simulink model "Zamora22210432HIPER"  (R2023a)
settings: Solver=ode15s  StartTime=0.0  StopTime=15  RelTol=1e-3
libraries: slpidlib x1
settings Model: Creator=Michelle  LastModifiedBy=Michelle
settings DataIOCC: ReturnWorkspaceOutputs=off  TimeSaveName=t
settings DebuggingCC: AlgebraicLoopMsg=none  ArtificialAlgebraicLoopMsg=none  MaxConsecutiveZCsMsg=none  InheritedTsInSrcMsg=none  MultiTaskCondExecSysMsg=none  MultiTaskRateTransMsg=warning  TasksWithSamePriorityMsg=none  SigSpecEnsureSampleTimeMsg=none  UnknownTsInhSupMsg=none  ModelReferenceExtraNoncontSigs=none  OperatingPointInterfaceChecksumMismatchMsg=none

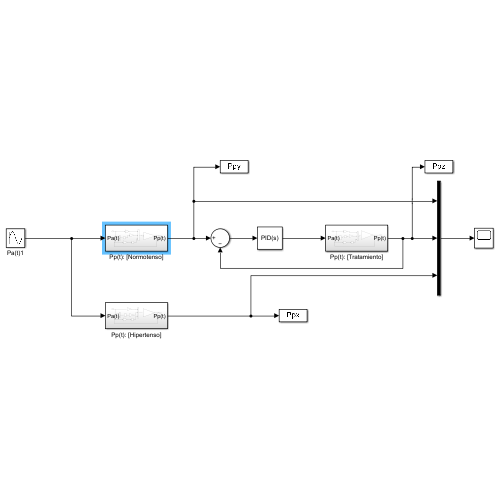
[thumbnail: Simulink's stored preview of the top-level diagram]
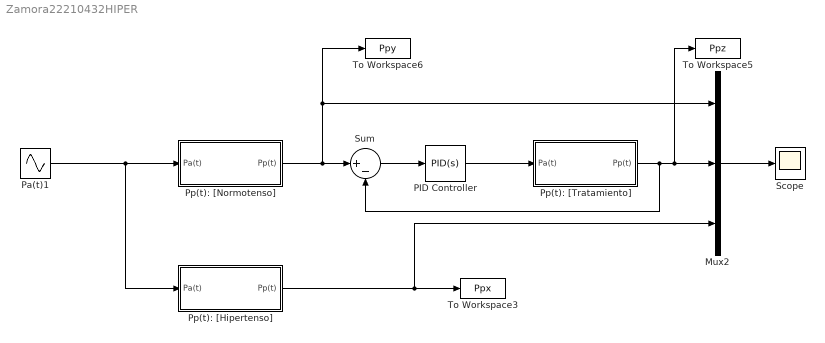
== system Zamora22210432HIPER ==
  Mux2 : Mux  Inputs=3
  PID Controller : slpidlib/PID Controller  Controller=PID  Form=Parallel  TimeDomain=Continuous-time  UseExternalTs=off  SampleTime=-1  IntegratorMethod=Forward Euler  FilterMethod=Forward Euler  ControllerParametersSource=internal  P=8.92851562535347e-05  I=1035.71406250139  UseKiTs=off  D=0  N=100  UseFilter=on  TunerSelectOption=Transfer Function Based (PID Tuner App)  InitialConditionSource=internal  InitialConditionForIntegrator=0  InitialConditionForFilter=0  DifferentiatorICPrevScaledInput=0  ExternalReset=none  TrackingMode=off  Kt=1  LimitOutput=off  SatLimitsSource=internal  UpperSaturationLimit=inf  LowerSaturationLimit=-inf  LinearizeAsGain=on  AntiWindupMode=none  Kb=1  LimitIntegrator=off  UpperIntegratorSaturationLimit=inf  LowerIntegratorSaturationLimit=-inf  POutMin=[]  POutMax=[]  IOutMin=[]  IOutMax=[]  DOutMin=[]  DOutMax=[]  NOutMin=[]  NOutMax=[]  SumOutMin=[]  SumOutMax=[]  SaturationOutMin=[]  SaturationOutMax=[]  PParamMin=[]  PParamMax=[]  IParamMin=[]  IParamMax=[]  DParamMin=[]  DParamMax=[]  NParamMin=[]  NParamMax=[]  KbParamMin=[]  KbParamMax=[]  KtParamMin=[]  KtParamMax=[]  KbOutMin=[]  KbOutMax=[]  KtOutMin=[]  KtOutMax=[]  IntegratorOutMin=[]  IntegratorOutMax=[]  FilterOutMin=[]  FilterOutMax=[]  SumI1OutMin=[]  SumI1OutMax=[]  SumI2OutMin=[]  SumI2OutMax=[]  SumI3OutMin=[]  SumI3OutMax=[]  SumI4OutMin=[]  SumI4OutMax=[]  SumDOutMin=[]  SumDOutMax=[]  DifferentiatorOutMin=[]  DifferentiatorOutMax=[]  FilterDiffOutCoefMin=[]  FilterDiffOutCoefMax=[]  ReciprocalOutMin=[]  ReciprocalOutMax=[]  SumDenOutMin=[]  SumDenOutMax=[]  SumNumOutMin=[]  SumNumOutMax=[]  DivideOutMin=[]  DivideOutMax=[]  UdiffTsProdOutMin=[]  UdiffTsProdOutMax=[]  NTsProdOutMin=[]  NTsProdOutMax=[]  UintegralTsProdOutMin=[]  UintegralTsProdOutMax=[]  UngainTsProdOutMin=[]  UngainTsProdOutMax=[]  ClampingZeroOutDataTypeStr=Inherit: Inherit via back propagation  ClampingZeroOutMin=[]  ClampingZeroOutMax=[]  FilterDenConstantOutDataTypeStr=Inherit: Inherit via back propagation  FilterDenConstantOutMin=[]  FilterDenConstantOutMax=[]  PCopyOutDataTypeStr=Inherit: Inherit via back propagation  PCopyOutMin=[]  PCopyOutMax=[]  NCopyOutDataTypeStr=Inherit: Inherit via back propagation  NCopyOutMin=[]  NCopyOutMax=[]  IntegratorContinuousStateAttributes=''  IntegratorStateMustResolveToSignalObject=off  IntegratorRTWStateStorageClass=Auto  FilterContinuousStateAttributes=''  FilterStateMustResolveToSignalObject=off  FilterRTWStateStorageClass=Auto  ParallelPVariant=InternalParameters  IdealPVariant=Disabled  IVariant=InternalParameters  DVariant=InternalParameters  IntegratorVariant=Continuous  SatVariant=Disabled  AWVariant=Passthrough  PCopyVariant=Disabled  TRVariant=Disabled  FdbkBlocksVariant=Forward  IdealPFdbkVariant=Disabled  SatFdbkVariant=Disabled  DerivativeFilterVariant=ContFilter  NVariant=InternalParameters  NCopyVariant=Disabled  FilterICVariant=InternalICsFilter  IntegratorICVariant=InternalICs  ExternalResetVariant=Disabled  TRSumVariant=Passthrough  SumFdbkVariant=Disabled  SumVariant=Sum_PID  TsampFilterVariant=InternalTs  TsampNgainVariant=Passthrough  TsampIntegralVariant=Disabled_SignalSpec  ExternalSaturationOutDataTypeStr=Inherit: Same as second input
  Pa(t)1 : Sin  Bias=0.8  Frequency=(2*pi)*(95/60)
  Pp(t): [Hipertenso] : Subsystem
  Pp(t): [Normotenso] : Subsystem
  Pp(t): [Tratamiento] : Subsystem
  Scope : Scope
  Sum : Sum  Inputs=|+-
  To Workspace3 : ToWorkspace  VariableName=Ppx  SampleTime=-1
  To Workspace5 : ToWorkspace  VariableName=Ppz  SampleTime=-1
  To Workspace6 : ToWorkspace  VariableName=Ppy  SampleTime=-1
  wires:
  Pp(t): [Tratamiento]/1(Pp(t)) -> Mux2/2, To Workspace5/1, Sum/2
  Mux2/1 -> Scope/1
  Pp(t): [Normotenso]/1(Pp(t)) -> Mux2/1, To Workspace6/1, Sum/1
  Sum/1 -> PID Controller/1
  Pp(t): [Hipertenso]/1(Pp(t)) -> Mux2/3, To Workspace3/1
  Pa(t)1/1 -> Pp(t): [Hipertenso]/1(Pa(t)), Pp(t): [Normotenso]/1(Pa(t))
  PID Controller/1 -> Pp(t): [Tratamiento]/1(Pa(t))

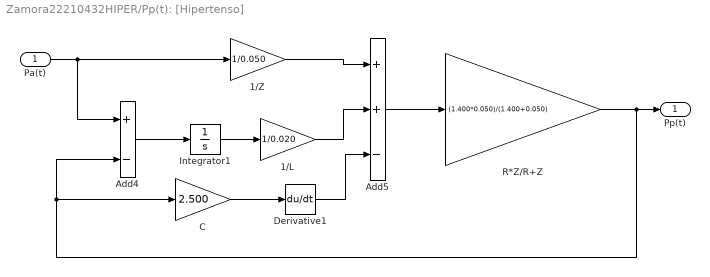
== system Zamora22210432HIPER/Pp(t): [Hipertenso] ==
  Pa(t) : Inport
  1/L : Gain  Gain=1/0.020
  1/Z : Gain  Gain=1/0.050
  Add4 : Sum  Inputs=+-
  Add5 : Sum  Inputs=++-
  C : Gain  Gain=2.500
  Derivative1 : Derivative
  Integrator1 : Integrator
  R*Z/R+Z : Gain  Gain=(1.400*0.050)/(1.400+0.050)
  Pp(t) : Outport  VectorParamsAs1DForOutWhenUnconnected=off
  wires:
  1/Z/1 -> Add5/1
  Derivative1/1 -> Add5/3
  C/1 -> Derivative1/1
  Add5/1 -> R*Z/R+Z/1
  Pa(t)/1 -> Add4/1, 1/Z/1
  R*Z/R+Z/1 -> C/1, Add4/2, Pp(t)/1
  Add4/1 -> Integrator1/1
  Integrator1/1 -> 1/L/1
  1/L/1 -> Add5/2

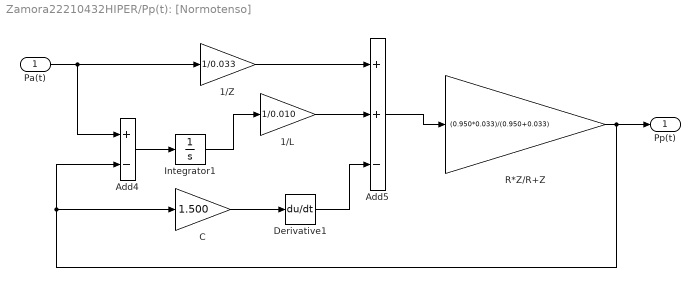
== system Zamora22210432HIPER/Pp(t): [Normotenso] ==
  Pa(t) : Inport
  1/L : Gain  Gain=1/0.010
  1/Z : Gain  Gain=1/0.033
  Add4 : Sum  Inputs=+-
  Add5 : Sum  Inputs=++-
  C : Gain  Gain=1.500
  Derivative1 : Derivative
  Integrator1 : Integrator
  R*Z/R+Z : Gain  Gain=(0.950*0.033)/(0.950+0.033)
  Pp(t) : Outport  VectorParamsAs1DForOutWhenUnconnected=off
  wires:
  1/Z/1 -> Add5/1
  Derivative1/1 -> Add5/3
  C/1 -> Derivative1/1
  Add5/1 -> R*Z/R+Z/1
  Pa(t)/1 -> Add4/1, 1/Z/1
  R*Z/R+Z/1 -> Pp(t)/1, C/1, Add4/2
  1/L/1 -> Add5/2
  Add4/1 -> Integrator1/1
  Integrator1/1 -> 1/L/1

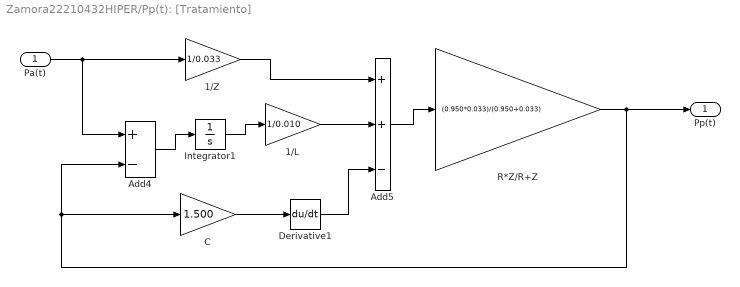
== system Zamora22210432HIPER/Pp(t): [Tratamiento] ==
  Pa(t) : Inport
  1/L : Gain  Gain=1/0.010
  1/Z : Gain  Gain=1/0.033
  Add4 : Sum  Inputs=+-
  Add5 : Sum  Inputs=++-
  C : Gain  Gain=1.500
  Derivative1 : Derivative
  Integrator1 : Integrator
  R*Z/R+Z : Gain  Gain=(0.950*0.033)/(0.950+0.033)
  Pp(t) : Outport  VectorParamsAs1DForOutWhenUnconnected=off
  wires:
  1/Z/1 -> Add5/1
  Derivative1/1 -> Add5/3
  C/1 -> Derivative1/1
  Add5/1 -> R*Z/R+Z/1
  Pa(t)/1 -> Add4/1, 1/Z/1
  R*Z/R+Z/1 -> Pp(t)/1, Add4/2, C/1
  1/L/1 -> Add5/2
  Integrator1/1 -> 1/L/1
  Add4/1 -> Integrator1/1
